simulink model "Throttle_Air_Mass_Flow"  (R2025b)
settings: Solver=VariableStepAuto  StartTime=0.0  StopTime=10.0  RelTol=1e-3
settings Model: Creator=Indo  LastModifiedBy=Indo

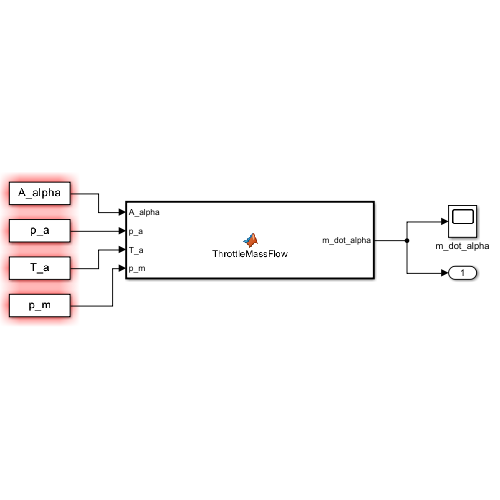
[thumbnail: Simulink's stored preview of the top-level diagram]
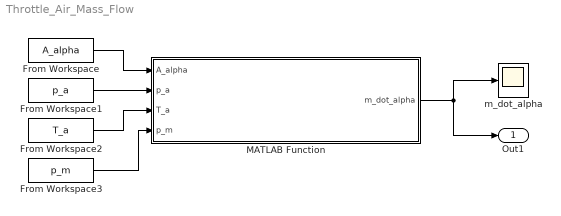
== system Throttle_Air_Mass_Flow ==
  From Workspace : FromWorkspace  VariableName=A_alpha
  From Workspace1 : FromWorkspace  VariableName=p_a
  From Workspace2 : FromWorkspace  VariableName=T_a
  From Workspace3 : FromWorkspace  VariableName=p_m
  MATLAB Function : MATLAB Function  TreatAsAtomicUnit=on
  m_dot_alpha : Scope
      settings: ActiveDisplayYMinimum=27272.349674040706  ActiveDisplayYMaximum=44653.278057688141
  Out1 : Outport
  wires:
  MATLAB Function/1(m_dot_alpha) -> m_dot_alpha/1, Out1/1
  From Workspace/1 -> MATLAB Function/1(A_alpha)
  From Workspace1/1 -> MATLAB Function/2(p_a)
  From Workspace2/1 -> MATLAB Function/3(T_a)
  From Workspace3/1 -> MATLAB Function/4(p_m)

== matlab function Throttle_Air_Mass_Flow/MATLAB Function ==
  data: A_alpha input; m_dot_alpha output; p_a input; T_a input; p_m input
function m_dot_alpha = ThrottleMassFlow(A_alpha, p_a, T_a, p_m)
% Throttle air mass flow
% A_alpha[m^2], p_a[Pa], T_a[K], p_m[Pa]
R = 287;                       % J/(kg·K)
r = p_m / p_a;
C = (A_alpha * p_a) / sqrt(R * T_a);
if r < 0.5
    m_dot_alpha = C * (1/sqrt(2));              % choked
else
    m_dot_alpha = C * sqrt(2*r*(1 - r));        % unchoked
end
end
